simulink model "PIDpodgrzewacz"  (R2015a)
settings: Solver=ode45  StartTime=0.0  StopTime=2000  FixedStep=0.001  RelTol=1e-3
values from neighbouring files (symbols this model uses):
  Kd = 20    [SilnikDC.m]    (also in funkcja.m = pid(2); funkcja1.m = pid(3); grzalka.m = output(3); grzałka.m = output(3))
  Ki = 200    [SilnikDC.m]    (also in funkcja.m = pid(3); funkcja1.m = pid(2); grzalka.m = output(2); grzałka.m = output(2))
  Kp = 100    [SilnikDC.m]    (also in funkcja.m = pid(1); funkcja1.m = pid(1); grzalka.m = output(1); grzałka.m = output(1))
  x = 1.0/11.2    (= 0.0892857142857)    [funkcja1.m]    (also in grzalka.m; grzałka.m)
  x1 = 1.0/(0.01*1000*4.19*1000.0)    (= 2.38663484487e-05)    [funkcja1.m]    (also in grzalka.m; grzałka.m)
  x2 = 0.0333*0.001*1000*4.19*1000.0    (= 139.527)    [funkcja1.m]    (also in grzalka.m; grzałka.m)
settings Model: Creator=Dawid  LastModifiedBy=Dawid

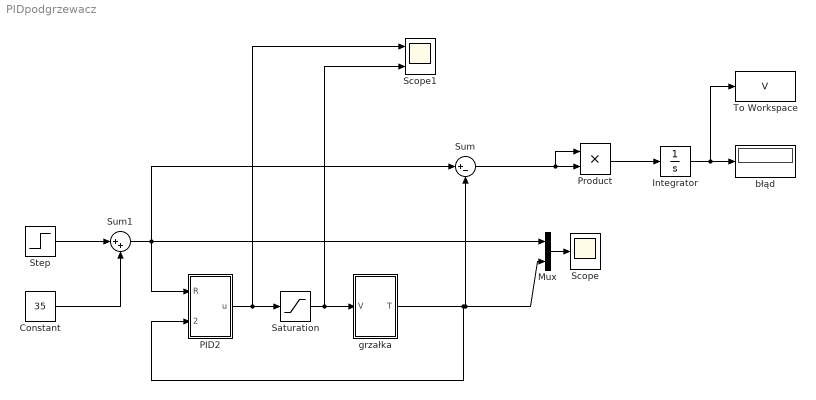
== system PIDpodgrzewacz ==
  Constant : Constant  Value=35
  Integrator : Integrator
  Mux : Mux  Inputs=2
  PID2 : Subsystem
  Product : Product
  Saturation : Saturate  UpperLimit=400  LowerLimit=0  ZeroCross=off
  Scope : Scope
      settings: TimeRange=4.302162424094797
  Scope1 : Scope  NumInputPorts=2
      settings: TimeRange=4.302162424094797  YMin=-5~-5  YMax=5~5
  Step : Step  Time=200  After=5  SampleTime=0
  Sum : Sum  Inputs=|+-
  Sum1 : Sum  Inputs=|++
  To Workspace : ToWorkspace  VariableName=V  SampleTime=-1
  "błąd " : Display
  "grzałka " : Subsystem
  wires:
  Sum/1 -> Product/1, Product/2
  Product/1 -> Integrator/1
  Integrator/1 -> To Workspace/1, "błąd "/1
  Step/1 -> Sum1/1
  Constant/1 -> Sum1/2
  Sum1/1 -> Mux/1, PID2/1("R "), Sum/1
  "grzałka "/1(T) -> Mux/2, Sum/2, PID2/2(speed)
  PID2/1(u) -> Scope1/1, Saturation/1
  Saturation/1 -> Scope1/2, "grzałka "/1("V ")
  Mux/1 -> Scope/1

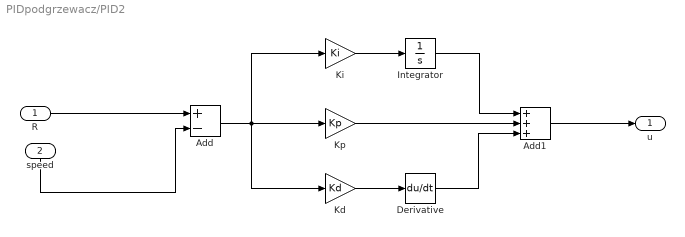
== system PIDpodgrzewacz/PID2 ==
  "R " : Inport
  speed : Inport  Port=2
  Add : Sum  Inputs=+-
  Add1 : Sum  Inputs=+++
  Derivative : Derivative
  Integrator : Integrator
  Kd : Gain  Gain=Kd
  "Ki " : Gain  Gain=Ki
  Kp : Gain  Gain=Kp
  u : Outport
  wires:
  Kp/1 -> Add1/2
  Integrator/1 -> Add1/1
  Kd/1 -> Derivative/1
  "Ki "/1 -> Integrator/1
  Add/1 -> Kd/1, "Ki "/1, Kp/1
  Add1/1 -> u/1
  Derivative/1 -> Add1/3
  "R "/1 -> Add/1
  speed/1 -> Add/2

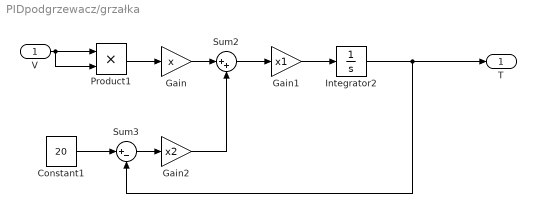
== system PIDpodgrzewacz/grzałka  ==
  "V " : Inport
  Constant1 : Constant  Value=20
  Gain : Gain  Gain=x
  Gain1 : Gain  Gain=x1
  Gain2 : Gain  Gain=x2
  Integrator2 : Integrator  InitialCondition=60
  Product1 : Product
  Sum2 : Sum  Inputs=|++
  Sum3 : Sum  Inputs=|+-
  T : Outport
  wires:
  Sum3/1 -> Gain2/1
  Sum2/1 -> Gain1/1
  Gain1/1 -> Integrator2/1
  Product1/1 -> Gain/1
  Gain/1 -> Sum2/1
  Gain2/1 -> Sum2/2
  Integrator2/1 -> T/1, Sum3/2
  Constant1/1 -> Sum3/1
  "V "/1 -> Product1/2, Product1/1
